simulink model "Virtual_Veh_Sim_EV3M_DLC"  (R2020a)
settings: configuration reference "Config_VarStep_Lat" (kept outside this file)
model workspace (MAT data in the model file):
  A = 159.22
  AccPwrbp = [0 0]
  AccSpdbp = [300 750]
  Aeff = 0.0314159265359
  Af = 2.46
  AfrStoich = 14.6
  AxlIxx = 62.3745166667
  AxlM = 160
  B = 1.01
  BattCapInit = 3.18
  BattCapInit_EV = 4.24
  BattChargeMax = 5.3
  BattChrgPwrMax = -60000
  BattChrgPwrMax_EV = -350000
  BattCurrMax = 300
  BattCurrMax_EV = 900
  BattDischrgPwrMax = 85000
  BattDischrgPwrMax_EV = 497000
  BattTempBp = [243.1 253.1 263.1 273.1 283.1 298.1 313.1]
  Battery.SOC_LUT = [0; 0.233616805137; 0.329414704495; 0.425212603853; 0.521010503211; 0.616808402569; 0.712606301927; 0.808404201284; 0.904202100642; 1]
  Battery.Temperature_LUT = [278.15 293.15 323.15]
  Battery.Capacity_LUT = [5.3 5.3 5.3]
  Battery.Em_LUT = [3.49587596064  3.51326111431  3.51592909009; 3.55858585798  3.5719535891  3.57237356974; 3.60724177033  3.62068327764  3.6276550187; 3.64771235788  3.65760001947  3.66611286097; 3.69314621195  3.69760962651  3.70681604299; 3.75549177279  3.75773263614  3.76696651763; 3.84165417727  3.85083489047  3.86645865382; 3.95105059257  3.95772489987  3.96617355496; 4.06366580695  4.067089232  4.07236317958; 4.1906518044  4.19061236732  4.19167206629]
  Battery.R0_LUT = [0.00999998116885  0.00969375106236  0.00708145896739; 0.00999856430024  0.00911239076326  0.00787358934878; 0.00998730272712  0.00894632530884  0.00837174615208; 0.00996262884044  0.00879430156772  0.00835611000801; 0.00987275439244  0.0083702809345  0.00820789809556; 0.00999543134051  0.00796657772792  0.0078372923375; 0.00990199705676  0.00829317762849  0.00843184907817; 0.00994753142013  0.00846223904615  0.00857747373973; 0.00988864262519  0.00860046339116  0.00783809261162; 0.00993546613466  0.00869430562795  0.00761030624168]
  Battery.R1_LUT = [0.00499947769959  0.00176414777168  0.00316403561543; 0.00499519961471  0.00182319958795  0.00222758288934; 0.00497942319098  0.00215602639557  0.00198515725158; 0.00498117211272  0.00190060293124  0.00183019810762; 0.00450940543796  0.0017898790503  0.00183803772559; 0.00398127966959  0.00191854781097  0.00207431379095; 0.00376691492773  0.00188008375757  0.00198672384849; 0.00419163622064  0.00214433717755  0.00161902199826; 0.00442604017912  0.00155246821646  0.0021103441137; 0.00431483823804  0.00154970784036  0.00218727749279]
  Battery.C1_LUT = [1983.38450838  78841.49366  1101.57625667; 4685.2948826  46429.6816213  4135.52830594; 9956.77541023  63356.4083796  12730.5976872; 11168.8695649  44437.7240428  12079.4670374; 4241.75396721  25121.8581323  9873.97196936; 4860.18499946  15430.1643159  2313.84302982; 8563.32887293  19567.7109152  8773.59604623; 11272.4596966  21732.1494006  11126.4679691; 3899.6527347  15798.9914071  2546.16773112; 2937.3854477  42171.3235856  1720.82916662]
  Battery.cell_mass = 0.066
  Battery.cell_rho_Cp = 2040000
  Battery.cell_Cp_heat = 964.92
  Battery.T_init = 288.15
  Battery.Qe_init = 1.06
  Battery.R_bleed = 20
  Battery.h_conv = 5
  Battery.cell_area = 0.1019
  Battery.TempInit = 298.15
  BrkPrsMax = 8273709
  Bx = 10
  C = 0.3618
  CapLUTBp = [0 0.01 0.02 0.03 0.04 0.05 0.06 0.07 0.08 0.09 0.1 0.11 0.12 0.13 0.14 0.15 0.16 0.17 0.18 0.19 0.2 0.21 0.22 0.23 0.24 0.25 0.26 0.27 0.28 0.29 0.3 0.31 0.32 0.33 0.34 0.35 0.36 0.37 0.38 0.39 0.4 0.41 0.42 0.43 0.44 0.45 0.46 0.47 0.48 0.49 0.5 0.51 0.52 0.53 0.54 0.55 0.56 0.57 0.58 0.59 0.6 0.61 0.62 0.63 0.64 0.65 0.66 0.67 0.68 0.69 0.7 0.71 0.72 0.73 0.74 0.75 0.76 0.77 0.78 0.79 0.8 0.81 0.82 0.83 0.84 0.85 0.86 0.87 0.88 0.89 0.9 0.91 0.92 0.93 0.94 0.95 0.96 0.97 0.98 0.99 1]
  CapSOCBp = [0 0.2 0.4 0.6 0.8 1]
  CatLightOffTime = 0
  Cd = 0.25
  ChrgLmt_bpt = [1 1 1 1 1 1 1 0.9 0.7 0.5 0]
  Cl = 0.1
  Cpm = 0.1
  Cps = 2
  CrankSpeed = 150
  Cx = 1.65
  Cz = 5565.2246438
  CzWhlAxl = 11490.971257
  DCT_Param.Transmission.Ratios = [3.78 2.18 1.43 1.03 0.935 0.84]
  DCT_Param.Transmission.Shaft_Inertia_Odd = 0.0023
  DCT_Param.Transmission.Shaft_Inertia_Even = 0.0009
  DCT_Param.Transmission.Shaft_Inertia_Output = 0.008
  DCT_Param.Transmission.Gear_Inertia = 0.001
  DCT_Param.Transmission.Gear_Efficiency = 0.94
  DCT_Param.Transmission.Gear_Ang_Vel_Thr = 0.01
  DCT_Param.Transmission.Shaft_Velocity_Odd = 0
  DCT_Param.Transmission.Shaft_Velocity_Even = 0
  DCT_Param.Transmission.Shaft_Velocity_Output = 0
  DCT_Param.Transmission.Gear_Initial_Velocity = 0
  DCT_Param.Transmission.Abstract.Compliance = 100000
  DCT_Param.Transmission.Abstract.Damping = 10000
  DCT_Param.Transmission.Abstract.Ratio_Time_Const = 0.05
  DCT_Param.Transmission.Abstract.Shift_Gear_Delay = 25
  DCT_Param.Clutch.Torque_Radius = 130
  DCT_Param.Clutch.Num_Friction_Surfaces = 4
  DCT_Param.Clutch.Engagement_Piston_Area = 0.001
  DCT_Param.Clutch.Kinetic_Friction_Coeff = 0.3
  DCT_Param.Clutch.Static_Friction_Coeff = 0.31
  DCT_Param.Clutch.Derating_Factor = 1
  DCT_Param.Clutch.Clutch_Velocity_Tolerance = 0.001
  DCT_Param.Clutch.Threshold_Pressure = 1
  DCT_Param.Clutch.Drag_Torque_Coeff = 0
  DCT_Param.Dog_Clutch.Max_Torque = 1000
  DCT_Param.Dog_Clutch.Teeth_Mean_Radius = 50
  DCT_Param.Dog_Clutch.Tooth_Height = 10
  DCT_Param.Dog_Clutch.Ring_Hub_Clearance = 3
  DCT_Param.Dog_Clutch.Ring_Stop_Stiffness = 1000000
  DCT_Param.Dog_Clutch.Ring_Stop_Damping = 1000
  DCT_Param.Dog_Clutch.Shift_Linkage_Damping = 100
  DCT_Param.Dog_Clutch.Max_Engage_Velocity = 1000000
  DCT_Param.Dog_Clutch.Tooth_Engage_Overlap = 3
  DCT_Param.Vehicle.Mass = 1600
  DCT_Param.Vehicle.Wheels_Per_Axle = 2
  DCT_Param.Vehicle.Distance_CG_FrontAxle = 1.7
  DCT_Param.Vehicle.Distance_CG_RearAxle = 2
  DCT_Param.Vehicle.Distance_CG_Ground = 0.5
  DCT_Param.Vehicle.Frontal_Area = 3
  DCT_Param.Vehicle.Aero_Drag_Coeff = 0.4
  DCT_Param.Vehicle.Initial_Velocity = 0
  DCT_Param.Vehicle.Final_Drive_Ratio = 3.7
  DCT_Param.Vehicle.Final_Drive_Efficiency = 0.86
  DCT_Param.Vehicle.Final_Drive_Vel_Thresh = 0.01
  DCT_Param.Vehicle.Side_Shaft_Inertia = 0.01
  DCT_Param.Vehicle.Side_Shaft_Initial_Velocity = 0
  DCT_Param.Vehicle.Tire.Radius = 0.312
  DCT_Param.Vehicle.Tire.Inertia = 0.5
  DCT_Param.Vehicle.Tire.Initial_Velocity = 0
  DCT_Param.Vehicle.Tire.Slip_Vel_Thresh = 0.1
  DCT_Param.Vehicle.Tire.Nominal_Vertical_Load = 4000
  DCT_Param.Vehicle.Tire.C_Coeff = 1.685
  DCT_Param.Vehicle.Tire.D_Coeff = [1.21 -0.037]
  DCT_Param.Vehicle.Tire.E_Coeff = [0.344 0.095 -0.02 0]
  DCT_Param.Vehicle.Tire.BCD_Coeff = [21.51 -0.163 0.245]
  DCT_Param.Vehicle.Tire.H_Coeff = [-0.002 0.002]
  DCT_Param.Vehicle.Tire.V_Coeff = [0 0]
  DCT_Param.ICE.Max_Power = 100000
  DCT_Param.ICE.Speed_At_Max_Power = 5500
  DCT_Param.ICE.Max_Speed = 7000
  DCT_Param.ICE.Stall_Speed = 200
  DCT_Param.ICE.Shaft_Inertia = 0.2
  DCT_Param.ICE.Initial_Velocity = 800
  DCT_Param.ICE.Idle_Ref_Spd = 800
  DCT_Param.ICE.Engine_Time_Constant = 0.2
  DCT_Param.ICE.Initial_Normalized_Throttle = 0
  DCT_Param.ICE.Speed_Threshold = 20
  DCT_Param.ICE.FC.Speed_Vector = [0 368.421052632 736.842105263 1105.26315789 1473.68421053 1842.10526316 2210.52631579 2578.94736842 2947.36842105 3315.78947368 3684.21052632 4052.63157895 4421.05263158 4789.47368421 5157.89473684 5526.31578947 5894.73684211 6263.15789474 6631.57894737 7000]
  DCT_Param.ICE.FC.Torque_Vector = [0 10.5263157895 21.0526315789 31.5789473684 42.1052631579 52.6315789474 63.1578947368 73.6842105263 84.2105263158 94.7368421053 105.263157895 115.789473684 126.315789474 136.842105263 147.368421053 157.894736842 168.421052632 178.947368421 189.473684211 200]
  DCT_Param.ICE.FC.Consumption_Table = [0.262945178015 0.225304787522 0.201465019624 0.191425874321 0.195187351614 0.212749451502 0.244112173984 0.289275519063 0.348239486736 0.421004077004 0.507569289868 0.607935125326 ... (400 elements, 20x20)]
  DCT_Param.Shift_Map_Example.Pedal_Positions = [0.1 0.4 0.5 0.9]
  DCT_Param.Shift_Map_Example.Upshift_Speeds = [11  20  26  34.5  43; 14  26  35  44.5  55; 17  31  42  52.5  65; 21  39  52  66.5  80]
  DCT_Param.Shift_Map_Example.Downshift_Speeds = [8.9  17  23.6  32.4  40.8; 11.5  22.7  32  41.6  52.2; 14  27  38.1  50  62; 18  33  48  62.6  76.2]
  DCT_Param.Shift_Map_ORIG.Pedal_Positions = [0.1 0.4 0.5 0.9]
  DCT_Param.Shift_Map_ORIG.Upshift_Speeds = [11.5  23.5  35.5  45.5  55.5; 14.5  26.5  38.5  48.5  58.5; 17.5  29.5  41.5  51.5  61.5; 20.5  32.5  44.5  54.5  64.5]
  DCT_Param.Shift_Map_ORIG.Downshift_Speeds = [8.5  20.5  32.5  42.5  52.5; 11.5  23.5  35.5  45.5  55.5; 14.5  26.5  38.5  48.5  58.5; 17.5  29.5  41.5  51.5  61.5]
  DCT_Param.Shift_Map_OPT.Pedal_Positions = [0.1 0.4 0.5 0.9]
  DCT_Param.Shift_Map_OPT.Upshift_Speeds = [17.8469  29.8469  35.8159  41.2981  46.3004; 19.2469  33.9778  43.9778  53.9778  63.9778; 24.5469  41.9778  62.1778  78.5778  106.9778; 27.5469  59.3778  99.0445  109.0445  119.0445]
  DCT_Param.Shift_Map_OPT.Downshift_Speeds = [14.8469  26.8469  32.8159  38.2981  43.3004; 16.2469  30.9778  40.9778  50.9778  60.9778; 21.5469  38.9778  59.1778  75.5778  103.9778; 24.5469  56.3778  96.0445  106.0445  116.0445]
  DCT_Param.Shift_Map.Pedal_Positions = [0.1 0.4 0.5 0.9]
  DCT_Param.Shift_Map.Upshift_Speeds = [11.5  23.5  35.5  45.5  55.5; 14.5  26.5  38.5  48.5  58.5; 17.5  29.5  41.5  51.5  61.5; 20.5  32.5  44.5  54.5  64.5]
  DCT_Param.Shift_Map.Downshift_Speeds = [8.5  20.5  32.5  42.5  52.5; 11.5  23.5  35.5  45.5  55.5; 14.5  26.5  38.5  48.5  58.5; 17.5  29.5  41.5  51.5  61.5]
  DCT_Param.Control.Clutch.Min_Lock_Pressure = 2000000
  DCT_Param.Control.Clutch.Max_Lock_Pressure = 5000000
  DCT_Param.Control.Clutch.Max_Unlock_Pressure = 500000
  DCT_Param.Control.Engine_Start_RPM = 800
  DCT_Param.Control.Engine_Stop_RPM = 790
  DCT_Param.Control.Mode_Logic_TS = 0.1
  DCT_Param.Control.ICE.Kp = 0.02
  DCT_Param.Control.ICE.Ki = 0.01
  DCT_Param.Control.Gen.Kp = 10
  DCT_Param.Control.Gen.Ki = 3
  DCT_Param.Control.Mot.Kp = 500
  DCT_Param.Control.Mot.Ki = 300
  DCT_Param.Control.Veh_Spd.Kp = 0.02
  DCT_Param.Control.Veh_Spd.Ki = 0.04
  DCT_Param.Driver.Kp = 400
  DCT_Param.Driver.Ki = 0.001
  DCT_Param.Driver.Pedal_Filter_Const = 0.01
  DCT_Param.Dog_Clutches.Pulse_Delay = 50
  DCT_Param.Dog_Clutches.Pulse_Length = 20
  DCT_Param.Animation.Teeth_Ratios = [0.338461538462 0.555555555556 0.916666666667 0.96 1.17948717949 1.92307692308]
  DCT_Param.Animation.Teeth_Ratios_Reverse = [0.458333333333 0.75]
  DCT_Param.Shift_Map_OPT506.Pedal_Positions = [0.1 0.4 0.5 0.9]
  DCT_Param.Shift_Map_OPT506.Upshift_Speeds = [18  30.2  48.3  67.3322  77.3429; 20.1  36.85  66.6178  76.7537  86.7537; 21.1  40.25  71.0189  81.0189  91.7873; 24.1  63.75  80.7523  105.9489  115.9489]
  DCT_Param.Shift_Map_OPT506.Downshift_Speeds = [15  27.2  45.3  64.3322  74.3429; 17.1  33.85  63.6178  73.7537  83.7537; 18.1  37.25  68.0189  78.0189  88.7873; 21.1  60.75  77.7523  102.9489  112.9489]
  DCT_Param.Shift_Map_OPTAbsRea176.Pedal_Positions = [0.1 0.4 0.5 0.9]
  DCT_Param.Shift_Map_OPTAbsRea176.Upshift_Speeds = [17.8469  29.8469  35.7875  44.0901  49.4243; 18.9219  34.1312  45.8256  59.7585  69.7585; 32.1719  43.4585  53.51  103.2151  114.6401; 35.1719  59.2585  99.5217  109.5217  119.5217]
  DCT_Param.Shift_Map_OPTAbsRea176.Downshift_Speeds = [14.8469  26.8469  32.7875  41.0901  46.4243; 15.9219  31.1312  42.8256  56.7585  66.7585; 29.1719  40.4585  50.51  100.2151  111.6401; 32.1719  56.2585  96.5217  106.5217  116.5217]
  DischrgLmt_bpt = [0 0.5 0.7 0.9 1 1 1 1 1 1 1]
  Dn_Shft_Spd = [3  7  11  15  19; 3  7  11  15  19; 10  17  26  35  49; 10  17  26  35  49]
  Downshift_Speeds = [9.5625  23.0625  36.5625  47.8125  59.0625  68.90625  78.75; 12.9375  26.4375  39.9375  51.1875  62.4375  72.84375  83.25; 16.3125  29.8125  43.3125  54.5625  65.8125  76.78125  87.75; 19.6875  33.1875  46.6875  57.9375  69.1875  80.71875  92.25]
  Dx = 1
  ECMS_Ki = 0.1
  ECMS_Kp = 3
  ECMS_method = 1
  ECMS_s = 3.4
  Em = [2.8 3.228 3.284 3.361 3.408 3.427 3.472 3.477 3.493 3.504 3.516 3.528 3.537 3.545 3.555 3.561 3.566 3.576 3.587 3.589 3.594 3.6 3.608 3.61 3.616 3.619 3.626 3.632 3.637 3.64 3.645 3.646 3.652 3.655 3.658 3.661 3.664 3.668 3.673 3.678 3.68 3.681 3.686 3.692 3.699 3.702 3.705 3.71 3.717 3.723 3.728 3.733 3.735 3.742 3.749 3.755 3.761 3.768 3.773 3.78 3.791 3.798 3.798 3.814 3.818 3.825 3.841 3.846 3.855 3.863 3.877 3.885 3.894 3.907 3.919 3.926 3.935 3.944 3.954 3.964 3.974 3.988 3.998 4.014 4.029 4.034 4.047 4.065 4.074 4.086 4.097 4.131 4.126 4.138 4.15 4.18 4.174 4.187 4.207 4.231 4.221]
  EngStopStartEnable = 1
  EngStopTime = Simulink.Parameter
  EngStopTime.Value = 0
  EngStopTime.DataType = 'auto'
  EngStopTime.Dimensions = [1 1]
  EngTrqCmd_0 = [0 5.91462851599 6.30130128159 6.63745773103 6.93103920513 7.1887141028 7.41614736865 7.6182009157 7.79908238179 7.96245469721 8.11151569725 8.24905488129 8.37749301819 8.49890935932 8.61506054978 8.72739478049 8.8370641951 8.94493799505 9.05161804887 9.15745812086 9.26258713198]
  Ex = 0.01
  F0z = [2886 2907]
  F0zWhlAxl = 2907
  FZMAX = 6570
  FZMIN = 0
  Fc = 500
  FsbF = [-700000 -7000 -700 0 700 7000 700000]
  FsbR = [-700000 -7000 -700 0 700 7000 700000]
  FskF = [-8928.57142857 -178.571428571 0 357.142857143 535.714285714 9285.71428571]
  FskR = [-5357.14285714 -107.142857143 0 214.285714286 321.428571429 5571.42857143]
  G = [-1 0 1 2 3 4 5 6]
  G_o = 1
  Gear_Dn_bpt = [2 3 4 5 6]
  Gear_Up_bpt = [1 2 3 4 5]
  HEVEngTrq_min = 16.186104388
  Hmax = 0.25
  Iyy = 3000
  Iyy_Whl = 0.8
  J = 0.01
  J1 = 0.01
  J2 = 0.01
  Jd = 0.025
  Ji = 0.1
  Jin = 0.05
  Jin_Cltch = 0.2
  Jin_Cltch2 = 0.01
  Jout = [0.01 0.009 0.01 0.01 0.01 0.01 0.01 0.01]
  Jout_Cltch = 0.01
  Jout_Cltch2 = 0.05
  Jt = 0.1
  Jw1 = 0.01
  Jw2 = 0.01
  K_c = 10000
  Kpt = 12798
  Kz = 52451.0065793
  KzWhlAxl = 138031.612078
  LHV = 43000000
  Lhv = 42940000
  Lrel = 0.15
  Mass = 1623
  MaxTorque = [10.8721902117; 76.2227873944; 95.7133163788; 115.203846226; 134.694376076; 154.184905918; 173.675435766; 181.839920951; 181.509869828; 181.17981871; 180.849767971; 180.519716854; 180.189665737; 179.859612653; 179.529561534; 179.199510415; 178.869460888; 178.539409771; 178.209357061; 177.879307536; 177.549246888]
  N = [3.39 1 4.212 2.637 1.8 1.386 1 0.772]
  NCyl = 4
  NF = 2
  NR = 2
  N_P0 = 3
  N_P4 = 4.1
  N_idle = 750
  Ndiff = 3.32
  Ndiff_P4 = 4.1
  Ndiff_front = 5
  Ndiff_rear = 3.5
  Ndisk = 1
  Ndisks = 4
  Ngrid = 200
  Np = 2
  Np_EV = 35
  Np_FC = 1
  Ns = 72
  Ns_EV = 96
  Pabs = 101325
  Pdl_Pos_Dn_bpt = [0 0.6 0.9 1]
  Pdl_Pos_Up_bpt = [0 0.25 0.9 1]
  Pedal_Positions = [0.1 0.4 0.5 0.9]
  PenaltyFctr = 10000000
  Plimit = 60000
  Plimit_EV = 350000
  Press = 7000000
  Pstd = 101325
  RInt = [0.008846  0.009319  0.009027  0.00847  0.01032  0.01314; 0.006389  0.006554  0.005553  0.005525  0.006043  0.007805; 0.004364  0.004101  0.00406  0.003452  0.003846  0.004517; 0.002031  0.002563  0.002532  0.00246  0.002716  0.003047; 0.001443  0.001825  0.001795  0.001778  0.001924  0.002234; 0.0005603  0.0007192  0.0006887  0.0007557  0.0007355  0.001014; 0.001028  0.001338  0.001  0.001536  0.001546  0.002789]
  Rair = 287
  Re = 0.327
  Reff = 0.11
  Reff_LSD = 0.2
  RegenBrkCutOff = [0 1]
  RegenBrkSpd_bpt = [2.2352 4.4704]
  Rm = 0.15
  SOCInit = 0.5
  SOCTrgt = 60
  SOC_bpt = [0 0.1 0.2 0.3 0.4 0.5 0.6 0.7 0.8 0.9 1]
  SOCmax = 80
  SOCmin = 40
  SUS.Zeta = 0.7071
  SUS.Wd = 9.42477796077
  SUS.Stiffness = 52451.0065793
  SUS.Damping.Constant = 5565.2246438
  SUS.UnsprungMass.Fr = 21.0693333333
  SUS.UnsprungMass.Rr = 21.0693333333
  Sg = 0.743
  Sinj = 6.45161290323
  T = 273
  TCopy = 300
  T_eff_bp = [0 20 40 60 80 100 120 140 160 180 200]
  T_eff_bp_EV_front = [0 30 60 90 120 150 180 210 240 270 300]
  T_eff_bp_EV_rear = [0 20 40 60 80 100 120 140 160 180 200]
  T_eff_bp_P0 = [0 5.78745247607 6.36619772368 7.07355302631 7.95774715459 9.09456817668 10.6103295395 12.7323954474 15.9154943092 21.2206590789 66.6666666667]
  T_init = 298.15
  T_t = [200 200 200 200 190.9859317 143.2394488 114.591559 95.49296586 81.85111359 71.61972439 63.66197724 57.29577951 52.08707228 47.74648293]
  T_t_EV_front = [300 300 300 300 286.47889755 214.8591732 171.8873385 143.23944879 122.776670385 107.429586585 95.49296586 85.943669265 78.13060842 71.619724395]
  T_t_EV_rear = [200 200 200 200 190.9859317 143.2394488 114.591559 95.49296586 81.85111359 71.61972439 63.66197724 57.29577951 52.08707228 47.74648293]
  T_t_P0 = [66.6666666667 66.6666666667 66.6666666667 66.6666666667 21.2206590789 15.9154943092 12.7323954474 10.6103295395 9.09456817668 7.95774715459 7.07355302631 6.36619772368 5.78745247607 5.30516476973]
  Tc_Batt = 0.001
  Tc_DC = 0.001
  Tc_Mot = 0.02
  Temp_bpts = [313 358]
  TimeCnstECP = 0.125
  TimeCnstEGR = 0.125
  TimeCnstETC = 0.085
  TimeCnstICP = 0.125
  TimeCnstIVL = 0.125
  TimeCnstMFA = 0.125
  TimeCnstSWVA = 0.125
  TimeCnstVCR = 0.125
  TimeCnstVGT = 0.15
  TimeCnstVIRL = 0.125
  TimeCnstWGA = 0.15
  TimeStep = 0.0001
  TracPenaltyFctr = 50
  Trans.InputShaftInertia = 0.01
  Trans.InputShaftDamping = 0.001
  Trans.FinalDrive = 2.77
  Trans.GearRatios = [-3.82 4.56 4.56 2.97 2.08 1.69 1.27 1 0.85 0.65]
  Trans.GearNums = [-1 0 1 2 3 4 5 6 7 8]
  Trans.Inertias = [0.128 0.01 0.128 0.1 0.062 0.028 0.01 0.01 0.01 0.01]
  Trans.DampingCoeffs = [0.003 0.001 0.003 0.0025 0.002 0.001 0.001 0.001 0.001 0.001]
  Trans.Efficiencies = [0.9 0.9 0.9 0.9 0.9 0.95 0.95 0.95 0.95 0.95]
  Trans.ShiftTau = 0.01
  Trq_bpts = [25 50 75 100 150 200 250]
  Ts = Simulink.Parameter
  Ts.Value = 0.01
  Ts.DataType = 'auto'
  Ts.Dimensions = [1 1]
  Tstd = 293.15
  UNLOADED_RADIUS = 0.336
  Up_Shft_Spd = [5  9  13  17  21; 5  9  13  17  21; 12  19  28  37  51; 12  19  28  37  51]
  Upshift_Speeds = [12.9375  26.4375  39.9375  51.1875  62.4375  72.84375  83.25; 16.3125  29.8125  43.3125  54.5625  65.8125  76.78125  87.75; 19.6875  33.1875  46.6875  57.9375  69.1875  80.71875  92.25; 33  52.5  77.25  100.5  138.75  161.875  185]
  VEH.Mass = 1181
  VEH.StaticNormalFrontLoad.FR = 264.666666667
  VEH.StaticNormalFrontLoad.FL = 264.666666667
  VEH.StaticNormalRearLoad.RR = 322
  VEH.StaticNormalRearLoad.RL = 322
  VEH.WheelBase = 3.075
  VEH.FrontAxlePositionfromCG = 1.515
  VEH.RearAxlePositionfromCG = 1.504
  VEH.HeightCG = 0.134
  VEH.FrontalArea = 2.11
  VEH.DragCoefficient = 0.33
  VEH.NumberOfWheelsPerAxle = 2
  VEH.Thread.FR = 1.705
  VEH.Thread.RR = 1.705
  VEH.PitchMomentInertia = 1922.66666667
  VEH.RollMomentInertia = 432.333333333
  VEH.YawMomentInertia = 2066
  VEH.SteeringRatio = 18
  VEH.TrackWidth = 1.922
  VEH.SprungMass = 1096.72266667
  VEH.InitialLongPosition = 0
  VEH.InitialLatPosition = 3.125
  VEH.InitialVertPosition = 0
  VEH.InitialRollAngle = 0
  VEH.InitialPitchAngle = 0
  VEH.InitialYawAngle = 0
  VEH.InitialLongVel = 0
  VEH.InitialLatVel = 0
  VEH.InitialVertVel = 0
  VEH.InitialRollRate = 0
  VEH.InitialPitchRate = 0
  VEH.InitialYawRate = 0
  VXLOW = 2
  Vd = 0.0015
  Vinit = 650
  WH.Mass = 11.4333333333
  a = 3
  aMy = 0.01
  a_CG = 1.09
  afr_stoich = 14.6
  alphaMy = 0
  b = Simulink.Parameter
  b.Value = 1000
  b.DataType = 'auto'
  b.Dimensions = [1 1]
  b1 = 100
  b1_g = 0.001
  b2 = 100
  b2_g = 0.001
  bMy = 0
  b_CG = 1.7
  b_J = 0.001
  bd = 0.001
  behavior = 0.2
  betaMy = 1
  bi = 0.001
  bin = 0.003
  bin_Cltch = 0.003
  bout = [0.003 0.003 0.003 0.003 0.003 0.003 0.003 0.003]
  bout_Cltch = 0.003
  br = 0.001
  bt = 0.001
  bw1 = 0.001
  bw2 = 0.001
  cMy = 0
  controller_type = 2
  defaultSpacing = 15
  disk_abore = 0.05
  domega_o = 0
  dt3D = 0.05
  dw = [0 10 20 40 60 80 100]
  dzdotsF = [-10 -1 -0.1 0 0.1 1 10]
  dzdotsR = [-10 -1 -0.1 0 0.1 1 10]
  dzsF = [-0.005 -0.0001 0 0.2 0.2001 0.2051]
  dzsR = [-0.005 -0.0001 0 0.2 0.2001 0.2051]
  eff = 98
  efficiency_table = [52  78  80  82  82  80  78  78  76  74  70; 52  78  80  82  82  80  78  78  76  74  70; 52  78  84  86  86  86  86  84  84  82  82; 52  80  86  86  88  88  88  86  86  84  84; 52  80  86  88  88  88  88  88  86  86  86; 52  80  86  88  90  90  90  90  88  88  88; 52  82  88  90  91  91  92  92  92  91  91; 52  82  88  91  91  92  93  93  93  93  93; 52  84  90  92  92  93  93  93  93  93  93; 62  86  91  93  93  93  93  93  93  93  93; 66  86  91  93  93  93  93  93  93  93  93; 70  86  92  93  93  93  93  93  93  93  93; 70  86  92  93  93  93  93  93  93  93  93; 72  86  91  93  93  93  93  93  93  93  93]
  efficiency_table_EV = [85  85  85  85  85  85  85  85  85  85  85; 85  85  90  90  90  90  90  90  90  90  88; 85  85  92  92  92  92  92  92  92  92  92; 85  85  92  92  93  93  93  93  92  92  92; 85  85  93  94  94  94  94  94  94  94  94; 85  85  93  94  94  95  95  95  95  95  95; 85  85  93  94  94  95  95  95  95  95  95; 85  85  93  94  95  95  95  95  95  95  95; 85  85  93  94  95  95  95  95  95  95  95; 85  85  93  94  94  94  94  94  94  94  94; 85  85  90  92  93  93  93  93  93  93  93; 85  85  90  92  93  93  93  93  93  93  93; 85  85  90  92  93  93  93  93  93  93  93; 85  85  90  92  93  93  93  93  93  93  93]
  efficiency_table_P0 = [52  78  80  82  82  80  78  78  76  74  70; 52  78  80  82  82  80  78  78  76  74  70; 52  78  84  86  86  86  86  84  84  82  82; 52  80  86  86  88  88  88  86  86  84  84; 52  80  86  88  88  88  88  88  86  86  86; 52  80  86  88  90  90  90  90  88  88  88; 52  82  88  90  91  91  92  92  92  91  91; 52  82  88  91  91  92  93  93  93  93  93; 52  84  90  92  92  93  93  93  93  93  93; 62  86  91  93  93  93  93  93  93  93  93; 66  86  91  93  93  93  93  93  93  93  93; 70  86  92  93  93  93  93  93  93  93  93; 70  86  92  93  93  93  93  93  93  93  93; 72  86  91  93  93  93  93  93  93  93  93]
  egotf = tf
  egotf.IOSize_ = [1 1]
  egotf.Data_ = ltipack.tfdata
  egotf.Data_.num = {[0 0 1]}
  egotf.Data_.den = {[0.5 1 0]}
  egotf.Data_.Delay.Input = 0
  egotf.Data_.Delay.Output = 0
  egotf.Data_.Delay.IO = 0
  egotf.Data_.Ts = 0
  elec_Pipe.Length = 75
  elec_Pipe.Dh = 2.5
  elec_Pipe.Area = 4.90873852123
  elec_Radiator.AreaG = 0.15
  elec_Radiator.VolumeG = 0.01
  elec_Radiator.AreaL = 0.000314159265359
  elec_Radiator.VolumeL = 0.000157079632679
  elec_Radiator.mdotG = [0.1 8]
  elec_Radiator.mdotL = [0.1 5]
  elec_Radiator.SD = [1  9; 2  10]
  elec_Radiator.dPG = [0.003 0.01]
  elec_Radiator.dPL = [0.005 0.02]
  eta = [0.95 0.95 0.95 0.95 0.95 0.95 0.95 0.95]
  eta_tbl = [0.7 0.8 0.9 0.9 0.9 0.9 0.9 0.7 0.8 0.9 0.9 0.9 ... (1232 elements, 7x11x8x2)]
  f_air = [0 0 0 0 0 0 0 0 0 0 0 0 ... (441 elements, 21x21)]
  f_co = [0 0 0 0 0 0 0 0 0 0 0 0 ... (441 elements, 21x21)]
  f_co2 = [0 0 0 0 0 0 0 0 0 0 0 0 ... (441 elements, 21x21)]
  f_cp_ld_bpt = [0 0.2 0.275 0.35 0.425 0.5 0.575 0.65 0.725 0.8 0.875 0.95 1.025 1.1 1.175 1.25]
  f_cp_n_bpt = [750 1053.57142857 1357.14285714 1660.71428571 1964.28571429 2267.85714286 2571.42857143 2875 3178.57142857 3482.14285714 3785.71428571 4089.28571429 4392.85714286 4696.42857143 5000]
  f_del_sa_bpt = [0 0.75 1.5 2.25 3 3.75 4.5 5.25 6 6.75 7.5 8.25 9 9.75 10.5 11.25 12 12.75 13.5 14.25 15 15.75 16.5 17.25 18 18.75 19.5 20.25 21 21.75 22.5 23.25 24 24.75 25.5 26.25 27 27.75 28.5 29.25 30 30.75 31.5 32.25 33 33.75 34.5 35.25 36 36.75 37.5 38.25 39 39.75 40.5 41.25 42 42.75 43.5 44.25 45 45.75 46.5 47.25 48]
  f_ecp = [0 0 7.19012817097 15.3709456879 19.1470470057 19.0854874367 13.5819971805 0 0 0 0 0 ... (240 elements, 16x15)]
  f_eff = [499.877436556 432.508206156 399.540781628 370.894662993 347.954880181 331.11554878 319.468905906 311.408898718 305.523567029 300.961538912 297.204959405 293.79866205 ... (441 elements, 21x21)]
  f_egr_areapct_cmd = [0 3.448 6.897 10.34 13.79 17.24 20.69 24.14 27.59 31.03 34.48 37.93 ... (600 elements, 30x20)]
  f_egr_areapct_nrmlzdflow_bpt = [0 0.03448 0.06897 0.1034 0.1379 0.1724 0.2069 0.2414 0.2759 0.3103 0.3448 0.3793 0.4138 0.4483 0.4828 0.5172 0.5517 0.5862 0.6207 0.6552 0.6897 0.7241 0.7586 0.7931 0.8276 0.8621 0.8966 0.931 0.9655 1]
  f_egr_areapct_pr_bpt = [0.5; 0.5263; 0.5526; 0.5789; 0.6053; 0.6316; 0.6579; 0.6842; 0.7105; 0.7368; 0.7632; 0.7895; 0.8158; 0.8421; 0.8684; 0.8947; 0.9211; 0.9474; 0.9737; 1]
  f_egr_max_stdflow = [74.87 74.87 74.74 74.39 73.81 72.98 71.91 70.58 68.97 67.06 64.84 62.25 59.27 55.81 51.79 47.07 36.33 24.22 12.11 0]
  f_egr_stdflow = [0 3.743 7.487 11.23 14.97 18.72 22.46 26.2 29.95 33.69 37.43 41.18 ... (420 elements, 21x20)]
  f_egr_stdflow_egrap_bpt = [0; 5; 10; 15; 20; 25; 30; 35; 40; 45; 50; 55; 60; 65; 70; 75; 80; 85; 90; 95; 100]
  f_egr_stdflow_pr_bpt = [0.5; 0.5263; 0.5526; 0.5789; 0.6053; 0.6316; 0.6579; 0.6842; 0.7105; 0.7368; 0.7632; 0.7895; 0.8158; 0.8421; 0.8684; 0.8947; 0.9211; 0.9474; 0.9737; 1]
  f_egrpct_cmd = [0  0  0  0  0  0  0  0  0  0  0  0  0  0  0; 0  0  0  0  0  0  0  0  0  0  0  0  0  0  0; 0  0  0  0  0  0  0  0  0  0  0  0  0  0  0; 0  0  0  0  0  0  0  0  0  0  0  0  0  0  0; 0  0  0  0  0  0  0  0  0  0  0  0  0  0  0; 0  0  0  0  0  0  0  0  0  0  0  0  0  0  0; 0  0  0  0  0  0  0  0  0  0  0  0  0  0  0; 0  0  0  0  0  0  0  0  0  0  0  0  0  0  0; 0  0  0  0  0  0  0  0  0  0  0  0  0  0  0; 0  0  0  0  0  0  0  0  0  0  0  0  0  0  0; 0  0  0  0  0  0  0  0  0  0  0  0  0  0  0; 0  0  0  0  0  0  0  0  0  0  0  0  0  0  0; 0  0  0  0  0  0  0  0  0  0  0  0  0  0  0; 0  0  0  0  0  0  0  0  0  0  0  0  0  0  0; 0  0  0  0  0  0  0  0  0  0  0  0  0  0  0; 0  0  0  0  0  0  0  0  0  0  0  0  0  0  0]
  f_egrpct_ld_bpt = [0 0.2 0.275 0.35 0.425 0.5 0.575 0.65 0.725 0.8 0.875 0.95 1.025 1.1 1.175 1.25]
  f_egrpct_n_bpt = [750 1054 1357 1661 1964 2268 2571 2875 3179 3482 3786 4089 4393 4696 5000]
  f_fric_temp_bpt = [275 277 279 281 283 285 287 289 291 293 295 297 299 301 303 305 307 309 311 313 315 317 319 321 323 325 327 329 331 333 335 337 339 341 343 345 347 349 351 353 355 357 359 361 363 365]
  f_fric_temp_mod = [3.986 2.616 2.132 1.946 1.839 1.747 1.672 1.608 1.551 1.499 1.462 1.415 1.363 1.314 1.275 1.248 1.223 1.195 1.173 1.15 1.134 1.113 1.097 1.082 1.065 1.051 1.039 1.025 1.01 1.001 0.9907 0.9802 0.9699 0.9595 0.9593 0.954 0.9415 0.9368 0.9285 0.923 0.9185 0.9093 0.9018 0.8989 0.8965 0.887]
  f_fuel = [0 0 0 0 0 0 0 0 0 0 0 0 ... (441 elements, 21x21)]
  f_hc = [0 0 0 0 0 0 0 0 0 0 0 0 ... (441 elements, 21x21)]
  f_icp = [0 0 1 1.09273642197 2.29409401139 3.54274371837 0.947749647567 0 0 0 0 0 ... (240 elements, 16x15)]
  f_intksys_stdflow_bpt = [0 29.67 59.34 89.01 117.8 144.1 155.7 166 175.2 183.3 190.7 197 202.7 207.7 212.2 216.1 219.4 222.2 224.5 226.4]
  f_intksys_stdflow_pr = [1 0.9789 0.9579 0.9368 0.9158 0.8947 0.8737 0.8526 0.8316 0.8105 0.7895 0.7684 0.7474 0.7263 0.7053 0.6842 0.6632 0.6421 0.6211 0.6]
  f_lamcmd = [1  1  1  1  1  1  1  1  1  1  1  1  1  1  1; 1  1  1  1  1  1  1  1  1  1  1  1  1  1  1; 1  1  1  1  1  1  1  1  1  1  1  1  1  1  1; 1  1  1  1  1  1  1  1  1  1  1  1  1  1  1; 1  1  1  1  1  1  1  1  1  1  1  1  1  1  1; 1  1  1  1  1  1  1  1  1  1  1  1  1  1  1; 1  1  1  1  1  1  1  1  1  1  1  1  1  1  1; 1  1  1  1  1  1  1  1  1  1  1  1  1  1  1; 1  1  1  1  1  1  1  1  1  1  1  1  1  1  1; 1  1  1  1  1  1  1  1  1  1  1  1  1  1  1; 1  1  1  1  1  1  1  1  1  1  1  1  1  1  0.978833376279; 1  1  1  1  1  0.994115442909  1  0.972947102204  0.980523305065  0.999379925377  1  0.999606769395  0.999730304812  0.995941175028  0.966904774685; 1  1  1  0.94651624294  1  0.952506105741  0.994491417815  0.906466250495  0.924122061249  0.974767007025  0.985748891861  0.982416523617  0.992900047913  0.942109771144  0.941787575943; 1  1  1  0.942  0.937279637266  0.910896768573  0.929830385386  0.839985398785  0.854904769548  0.889462296842  0.92380217143  0.919912974116  0.958707785886  0.945711085936  0.914402970615; 1  1  1  0.942  0.902  0.869287431405  0.865169352957  0.81  0.824  0.812  0.837314196571  0.85940898562  0.888506841156  0.882667105929  0.87548189152; 1  1  1  0.942  0.902  0.846  0.824  0.81  0.824  0.812  0.826  0.818  0.815209011399  0.813810193086  0.836]
  f_lamcmd_ld_bpt = [0 0.2 0.275 0.35 0.425 0.5 0.575 0.65 0.725 0.8 0.875 0.95 1.025 1.1 1.175 1.25]
  f_lamcmd_n_bpt = [750 1053.57142857 1357.14285714 1660.71428571 1964.28571429 2267.85714286 2571.42857143 2875 3178.57142857 3482.14285714 3785.71428571 4089.28571429 4392.85714286 4696.42857143 5000]
  f_lcmd = [0 0.323404450126 0.402272754123 0.472190900601 0.545782048677 0.619112163094 0.619299299836 0.619299299836 0.619299299836 0.619299299836 0.619299299836 0.619299299836 ... (315 elements, 21x15)]
  f_lcmd_n_bpt = [750 1053.57142857 1357.14285714 1660.71428571 1964.28571429 2267.85714286 2571.42857143 2875 3178.57142857 3482.14285714 3785.71428571 4089.28571429 4392.85714286 4696.42857143 5000]
  f_lcmd_tq_bpt = [0 15 25.2631578947 35.5263157895 45.7894736842 56.0526315789 66.3157894737 76.5789473684 86.8421052632 97.1052631579 107.368421053 117.631578947 127.894736842 138.157894737 148.421052632 158.684210526 168.947368421 179.210526316 189.473684211 199.736842105 210]
  f_m_lam = [0.94128 0.95565 0.97001 0.98437 0.99008 1.0004 0.97527 0.9549 0.92612 0.89735]
  f_m_lam_bpt = [0.65 0.7 0.75 0.8 0.85 0.9 0.95 1 1.05 1.1]
  f_m_sa = [1.0019 0.9988 0.9953 0.99173 0.98811 0.98441 0.98065 0.97682 0.97293 0.96897 0.96493 0.96083 0.95666 0.95242 0.94811 0.94373 0.93927 0.93475 0.93015 0.92548 0.92074 0.91592 0.91104 0.90608 0.90105 0.89594 0.89076 0.88551 0.88019 0.8748 0.86933 0.86379 0.85818 0.8525 0.84675 0.84093 0.83503 0.82907 0.82303 0.81693 0.81075 0.80451 0.79819 0.79181 0.78536 0.77884 0.77226 0.7656 0.75888 0.75209 0.74524 0.73832 0.73134 0.72429 0.71717 0.70999 0.70275 0.69682 0.68949 0.68303 0.67548 0.67037 0.66525 0.66014 0.65503]
  f_mdot_air_corr = [1.02156051768 1.00597426471 0.989411677851 1.0033499089 0.984591437857 0.988509040623 1.0326198627 1.02765527362 1.0134784519 0.998280021213 0.981755128787 0.967218261288 ... (400 elements, 20x20)]
  f_mdot_air_corr_ld_bpt = [0.223381333333 0.285105122807 0.346828912281 0.408552701754 0.470276491228 0.532000280702 0.593724070175 0.655447859649 0.717171649123 0.778895438596 0.84061922807 0.902343017544 0.964066807018 1.02579059649 1.08751438596 1.14923817544 1.21096196491 1.27268575439 1.33440954386 1.39613333333]
  f_mdot_air_n_bpt = [750 973.6842 1197.3684 1421.0526 1644.7368 1868.4211 2092.1053 2315.7895 2539.4737 2763.1579 2986.8421 3210.5263 3434.2105 3657.8947 3881.5789 4105.2632 4328.9474 4552.6316 4776.3158 5000]
  f_mdot_intk = [0 0 0 0 0 0 0 0 0 0 0 0 ... (400 elements, 20x20)]
  f_mdot_intk_ecp_bpt = [0 2.6316 5.2632 7.8947 10.5263 13.1579 15.7895 18.4211 21.0526 23.6842 26.3158 28.9474 31.5789 34.2105 36.8421 39.4737 42.1053 44.7368 47.3684 50]
  f_mdot_trpd_bpt = [0 5.7895 11.5789 17.3684 23.1579 28.9474 34.7368 40.5263 46.3158 52.1053 57.8947 63.6842 69.4737 75.2632 81.0526 86.8421 92.6316 98.4211 104.2105 110]
  f_nox = [0 0 0 0 0 0 0 0 0 0 0 0 ... (441 elements, 21x21)]
  f_nv = [0.64175366561 0.641419295169 0.640125365558 0.638690556197 0.644169906538 0.669178791311 0.731659452876 0.750078238889 0.750078238889 0.750078238889 0.750078238889 0.750078238889 ... (225 elements, 15x15)]
  f_nv_n_bpt = [750 1053.57142857 1357.14285714 1660.71428571 1964.28571429 2267.85714286 2571.42857143 2875 3178.57142857 3482.14285714 3785.71428571 4089.28571429 4392.85714286 4696.42857143 5000]
  f_nv_prs_bpt = [31 40.6428571429 50.2857142857 59.9285714286 69.5714285714 79.2142857143 88.8571428571 98.5 108.142857143 117.785714286 127.428571429 137.071428571 146.714285714 156.357142857 166]
  f_pm = [0  0  0  0  0  0  0  0  0  0  0  0  0  0  0  0  0  0  0  0  0; 0  0  0  0  0  0  0  0  0  0  0  0  0  0  0  0  0  0  0  0  0; 0  0  0  0  0  0  0  0  0  0  0  0  0  0  0  0  0  0  0  0  0; 0  0  0  0  0  0  0  0  0  0  0  0  0  0  0  0  0  0  0  0  0; 0  0  0  0  0  0  0  0  0  0  0  0  0  0  0  0  0  0  0  0  0; 0  0  0  0  0  0  0  0  0  0  0  0  0  0  0  0  0  0  0  0  0; 0  0  0  0  0  0  0  0  0  0  0  0  0  0  0  0  0  0  0  0  0; 0  0  0  0  0  0  0  0  0  0  0  0  0  0  0  0  0  0  0  0  0; 0  0  0  0  0  0  0  0  0  0  0  0  0  0  0  0  0  0  0  0  0; 0  0  0  0  0  0  0  0  0  0  0  0  0  0  0  0  0  0  0  0  0; 0  0  0  0  0  0  0  0  0  0  0  0  0  0  0  0  0  0  0  0  0; 0  0  0  0  0  0  0  0  0  0  0  0  0  0  0  0  0  0  0  0  0; 0  0  0  0  0  0  0  0  0  0  0  0  0  0  0  0  0  0  0  0  0; 0  0  0  0  0  0  0  0  0  0  0  0  0  0  0  0  0  0  0  0  0; 0  0  0  0  0  0  0  0  0  0  0  0  0  0  0  0  0  0  0  0  0; 0  0  0  0  0  0  0  0  0  0  0  0  0  0  0  0  0  0  0  0  0; 0  0  0  0  0  0  0  0  0  0  0  0  0  0  0  0  0  0  0  0  0; 0  0  0  0  0  0  0  0  0  0  0  0  0  0  0  0  0  0  0  0  0; 0  0  0  0  0  0  0  0  0  0  0  0  0  0  0  0  0  0  0  0  0; 0  0  0  0  0  0  0  0  0  0  0  0  0  0  0  0  0  0  0  0  0; 0  0  0  0  0  0  0  0  0  0  0  0  0  0  0  0  0  0  0  0  0]
  f_sa = [9.05 9.05 16.4373253582 15.3405265461 13.6074880273 9.83352189562 3.89388784387 0 0 0 0 0 ... (240 elements, 16x15)]
  f_sa_ld_bpt = [0 0.2 0.275 0.35 0.425 0.5 0.575 0.65 0.725 0.8 0.875 0.95 1.025 1.1 1.175 1.25]
  f_sa_n_bpt = [750 1053.57142857 1357.14285714 1660.71428571 1964.28571429 2267.85714286 2571.42857143 2875 3178.57142857 3482.14285714 3785.71428571 4089.28571429 4392.85714286 4696.42857143 5000]
  f_sa_opt = [35.3085 21.0105 10.3714 8.5076 7.1426 7.5656 -5.7766 -16.7061 -16.8345 -19.3546 -20.6085 -22.0872 ... (225 elements, 15x15)]
  f_startup_ect_bpt = [-40 0 20 50]
  f_startup_lambda_delta = [0.5 0.3 0.2 0]
  f_startup_lambda_delta_timecnst = [90 40 12 0]
  f_susp_axl_bp = [1 2]
  f_susp_dz_bp = [-0.325022776267 -0.315022776267 -0.305022776267 -0.205022776267 -0.105022776267 -0.00502277626717 0.0949772237328 0.194977223733 0.204977223733 0.214977223733]
  f_susp_dzdot_bp = [-3 -0.3 -0.2 -0.1 0 0.1 0.2 0.3 3]
  f_susp_fmz = [-144070.391448 -93629.24037 -75929.1118915 -20630.5828179 -15385.48216 -10140.3815021 -4895.28084414 349.819813785 -31916.3973792 18437.6709544 -83996.1993354 -33555.0482577 ... (43920 elements, 10x9x61x2x4)]
  f_susp_geom = [0 0 0 0 0 0 0 0 0 0 0 0 ... (3660 elements, 10x61x2x3)]
  f_susp_strgdelta_bp = [-0.523598775598 -0.506145483078 -0.488692190558 -0.471238898038 -0.453785605519 -0.436332312999 -0.418879020479 -0.401425727959 -0.383972435439 -0.366519142919 -0.349065850399 -0.331612557879 -0.314159265359 -0.296705972839 -0.279252680319 -0.261799387799 -0.244346095279 -0.226892802759 -0.209439510239 -0.191986217719 -0.174532925199 -0.157079632679 -0.13962634016 -0.12217304764 -0.10471975512 -0.0872664625997 -0.0698131700798 -0.0523598775598 -0.0349065850399 -0.0174532925199 0 0.0174532925199 0.0349065850399 0.0523598775598 0.0698131700798 0.0872664625997 0.10471975512 0.12217304764 0.13962634016 0.157079632679 0.174532925199 0.191986217719 0.209439510239 0.226892802759 0.244346095279 0.261799387799 0.279252680319 0.296705972839 0.314159265359 0.331612557879 0.349065850399 0.366519142919 0.383972435439 0.401425727959 0.418879020479 0.436332312999 0.453785605519 0.471238898038 0.488692190558 0.506145483078 0.523598775598]
  f_t_exh = [739.936218766 750.584766028 772.770773797 791.235245621 803.106549716 885.862998064 920.498479307 920.498479307 920.498479307 920.498479307 920.498479307 920.498479307 ... (225 elements, 15x15)]
  f_t_exh_l_bpt = [0.2 0.275 0.35 0.425 0.5 0.575 0.65 0.725 0.8 0.875 0.95 1.025 1.1 1.175 1.25]
  f_t_exh_n_bpt = [750 1053.57142857 1357.14285714 1660.71428571 1964.28571429 2267.85714286 2571.42857143 2875 3178.57142857 3482.14285714 3785.71428571 4089.28571429 4392.85714286 4696.42857143 5000]
  f_tap = [0 0.9375 0.9375 0.982121188204 1.22093639741 1.5421156717 1.98870690459 2.59666257968 2.6875 2.6875 2.6875 2.6875 ... (315 elements, 21x15)]
  f_tap_ld_bpt = [0 0.2 0.268421052632 0.336842105263 0.405263157895 0.473684210526 0.542105263158 0.610526315789 0.678947368421 0.747368421053 0.815789473684 0.884210526316 0.952631578947 1.02105263158 1.08947368421 1.15789473684 1.22631578947 1.29473684211 1.36315789474 1.43157894737 1.5]
  f_tap_n_bpt = [750 1053.57142857 1357.14285714 1660.71428571 1964.28571429 2267.85714286 2571.42857143 2875 3178.57142857 3482.14285714 3785.71428571 4089.28571429 4392.85714286 4696.42857143 5000]
  f_tbrake = [0 10.8721902117 10.8721902117 10.8721902117 10.8721902117 10.8721902117 10.8721902117 10.8721902117 10.8721902117 10.8721902117 10.8721902117 10.8721902117 ... (441 elements, 21x21)]
  f_tbrake_n_bpt = [0 750 973.684210526 1197.36842105 1421.05263158 1644.73684211 1868.42105263 2092.10526316 2315.78947368 2539.47368421 2763.15789474 2986.84210526 3210.52631579 3434.21052632 3657.89473684 3881.57894737 4105.26315789 4328.94736842 4552.63157895 4776.31578947 5000]
  f_tbrake_t_bpt = [0; 16.186104388; 24.9146526824; 33.6432009767; 42.3717492711; 51.1002975655; 59.8288458599; 68.5573941543; 77.2859424487; 86.0144907431; 94.7430390375; 103.471587332; 112.200135626; 120.928683921; 129.657232215; 138.385780509; 147.114328804; 155.842877098; 164.571425393; 173.299973687; 182.028521981]
  f_texh = [630.359790352 638.212816583 644.85156876 656.410931683 676.180276582 706.880985433 749.880156186 804.757804763 869.00210738 938.264388175 1007.38061415 1071.70023123 ... (441 elements, 21x21)]
  f_tm_corr = [0.839360054391 0.833393271885 0.82629554201 0.818442814437 0.811524387436 0.809164184856 0.814606352881 0.826887956871 0.842304598924 0.856886829014 0.869487025783 0.880530414174 ... (400 elements, 20x20)]
  f_tm_corr_n_bpt = [750 973.6842 1197.3684 1421.0526 1644.7368 1868.4211 2092.1053 2315.7895 2539.4737 2763.1579 2986.8421 3210.5263 3434.2105 3657.8947 3881.5789 4105.2632 4328.9474 4552.6316 4776.3158 5000]
  f_tm_corr_nd_bpt = [0.3 0.38947 0.47895 0.56842 0.65789 0.74737 0.83684 0.92632 1.0158 1.1053 1.1947 1.2842 1.3737 1.4632 1.5526 1.6421 1.7316 1.8211 1.9105 2]
  f_tpp = [0 100]
  f_tpp_tap_bpt = [0 100]
  f_tq_fric = [4.16  4.8  5.44  6.05  6.64  7.23  7.81  8.39  8.97  9.54  10.1  10.7  11.3  11.9  12.5; 4.42  5.07  5.69  6.29  6.89  7.49  8.09  8.69  9.28  9.86  10.4  11  11.6  12.2  12.8; 4.69  5.36  5.98  6.58  7.18  7.79  8.41  9.02  9.62  10.2  10.8  11.4  11.9  12.5  13.1; 4.88  5.59  6.25  6.87  7.48  8.09  8.71  9.32  9.92  10.5  11.1  11.7  12.3  12.9  13.4; 4.94  5.74  6.45  7.12  7.75  8.37  8.99  9.59  10.2  10.8  11.4  11.9  12.6  13.2  13.8; 4.93  5.76  6.56  7.29  7.97  8.62  9.23  9.83  10.4  11  11.6  12.2  12.8  13.4  14.1; 4.85  5.67  6.57  7.37  8.11  8.8  9.43  10  10.6  11.2  11.8  12.4  13  13.7  14.3; 4.74  5.57  6.46  7.34  8.14  8.88  9.55  10.2  10.8  11.4  12  12.6  13.2  13.8  14.4; 4.63  5.42  6.27  7.19  8.05  8.83  9.55  10.2  10.9  11.5  12.1  12.7  13.3  14  14.6; 4.52  5.29  6.11  6.98  7.84  8.65  9.4  10.1  10.8  11.5  12.1  12.8  13.4  14.1  14.6; 4.42  5.18  5.97  6.79  7.6  8.39  9.15  9.88  10.6  11.3  12.1  12.8  13.5  14.1  14.7; 4.34  5.09  5.86  6.64  7.42  8.17  8.88  9.6  10.3  11.1  11.9  12.7  13.4  14.1  14.7; 4.27  5.01  5.76  6.52  7.28  8.03  8.74  9.39  10.1  10.8  11.6  12.4  13.2  14  14.7; 4.21  4.94  5.67  6.42  7.16  7.89  8.59  9.25  9.93  10.7  11.5  12.3  13.1  13.8  14.6; 4.15  4.87  5.6  6.33  7.06  7.77  8.47  9.14  9.84  10.6  11.3  12.1  12.9  13.7  14.4]
  f_tq_inr = [25.8508 37.8267 50.6081 62.6825 74.6026 88.9064 81.9508 76.6399 82.9886 85.0042 88.9209 92.7645 ... (225 elements, 15x15)]
  f_tq_inr_l_bpt = [0.2 0.28571 0.37143 0.45714 0.54286 0.62857 0.71429 0.8 0.88571 0.97143 1.0571 1.1429 1.2286 1.3143 1.4]
  f_tq_inr_n_bpt = [750 1053.5714 1357.1429 1660.7143 1964.2857 2267.8571 2571.4286 2875 3178.5714 3482.1429 3785.7143 4089.2857 4392.8571 4696.4286 5000]
  f_tq_nl = [0 15.0012133443 26.4298333923 37.8556656512 49.2846782956 60.7113978793 72.3451969202 77.459652163 78.5324534074 78.5324534074 78.5324534074 78.5324534074 ... (256 elements, 16x16)]
  f_tq_nl_l_bpt = [0 0.2 0.275 0.35 0.425 0.5 0.575 0.65 0.725 0.8 0.875 0.95 1.025 1.1 1.175 1.25]
  f_tq_nl_n_bpt = [0 750 1053.57142857 1357.14285714 1660.71428571 1964.28571429 2267.85714286 2571.42857143 2875 3178.57142857 3482.14285714 3785.71428571 4089.28571429 4392.85714286 4696.42857143 5000]
  f_tq_pump = [7.24  7.7  7.82  7.95  8.1  8.27  8.45  8.64  8.78  8.88  8.96  9.03  9.12  9.25  9.45; 5.67  6.03  6.37  6.67  6.92  7.14  7.33  7.5  7.67  7.84  8.01  8.19  8.38  8.58  8.8; 3.94  4.52  5  5.36  5.6  5.77  5.92  6.1  6.35  6.67  7.02  7.4  7.75  8.06  8.34; 2.59  3.14  3.57  3.86  4.05  4.21  4.43  4.76  5.21  5.75  6.32  6.85  7.3  7.65  7.92; 1.8  2.25  2.61  2.88  3.11  3.37  3.71  4.17  4.74  5.36  5.96  6.49  6.91  7.23  7.46; 1  1.36  1.77  2.15  2.51  2.88  3.31  3.8  4.37  4.98  5.57  6.11  6.57  6.94  7.25; 1  1  1  1.09  1.59  2.08  2.6  3.17  3.81  4.49  5.19  5.85  6.44  6.92  7.29; 1  1  1  1  1  1.62  2.32  3.05  3.83  4.64  5.44  6.19  6.82  7.31  7.65; 1  1  1  1  1  1.35  2.21  3.08  3.97  4.88  5.78  6.64  7.41  8.06  8.58; 1  1  1  1  1  1  1.77  2.67  3.58  4.55  5.6  6.73  7.91  9.07  10.1; 1  1  1  1  1  1  1.72  2.67  3.61  4.62  5.79  7.15  8.69  10.3  11.9; 1  1  1  1  1  1  1.74  2.88  3.96  5.08  6.36  7.86  9.57  11.4  13.2; 1  1  1  1  1  1  1.37  2.7  4.01  5.39  6.92  8.65  10.5  12.4  14.2; 1  1  1  1  1  1  1.28  2.66  4.14  5.72  7.43  9.28  11.2  13.1  14.8; 1  1  1  1  1  1  1.39  2.82  4.39  6.06  7.85  9.73  11.6  13.5  15.1]
  f_twc_eff_co = [0.17 0.25 0.45 0.99 0.99 0.99 0.99]
  f_twc_eff_hc = [0.21 0.375 0.75 0.98 0.98 0.98 0.98]
  f_twc_eff_lam = [0.909090909 0.944055944 0.979020979 1 1.013986014 1.048951049 1.083916084]
  f_twc_eff_nox = [0.98 0.98 0.98 0.97 0.05 0.02 0]
  f_vivc = [0.37716 0.38164 0.38611 0.39033 0.39428 0.39795 0.40132 0.40441 0.40719 0.40967 0.41184 0.41372 0.41529 0.41656 0.41755 0.41825 0.41867 0.41884 0.41874 0.41865]
  f_vivc_icp_bpt = [0 2.6316 5.2632 7.8947 10.5263 13.1579 15.7895 18.4211 21.0526 23.6842 26.3158 28.9474 31.5789 34.2105 36.8421 39.4737 42.1053 44.7368 47.3684 50]
  f_wap = [100 100 100 100 100 100 100 99.9999999843 99.9999999843 99.9999999843 99.9999999843 99.9999999843 ... (315 elements, 21x15)]
  f_wap_ld_bpt = [0 0.2 0.268421052632 0.336842105263 0.405263157895 0.473684210526 0.542105263158 0.610526315789 0.678947368421 0.747368421053 0.815789473684 0.884210526316 0.952631578947 1.02105263158 1.08947368421 1.15789473684 1.22631578947 1.29473684211 1.36315789474 1.43157894737 1.5]
  f_wap_n_bpt = [750 1053.57142857 1357.14285714 1660.71428571 1964.28571429 2267.85714286 2571.42857143 2875 3178.57142857 3482.14285714 3785.71428571 4089.28571429 4392.85714286 4696.42857143 5000]
  g = 9.81
  h = 0.134
  k = Simulink.Parameter
  k.Value = 10000
  k.DataType = 'auto'
  k.Dimensions = [1 1]
  k1 = 50000
  k2 = 50000
  kappamax = 1.5
  lam_x = 1
  maxAccel = 3
  maxVel = 20
  minAccel = -3
  mu_kinetic = 0.35
  mu_static = 0.45
  muc = [0.16 0.13 0.115 0.11 0.105 0.1025 0.10125]
  muk = 0.4
  mus = 0.45
  numWheel = 4
  num_pads = 2
  omega1_c = 3000
  omega2_c = 3000
  omega_bpts = [52.4 78.5 105 131 157 183 209 262 314 419 524]
  omega_c = Simulink.Parameter
  omega_c.Value = 500
  omega_c.DataType = 'auto'
  omega_c.Dimensions = [1 1]
  omega_o = 0
  omega_o_J = 0
  omegai_o = 0
  omegain_o = 0
  omegal = 94.2477796077
  omegao = 0
  omegaout_o = 0
  omegat_o = 0
  omegau = 83.7758040957
  omegaw1o = 0
  omegaw2o = 0
  phi = [0 0.5 0.6 0.7 0.8 0.87 0.92 0.94 0.96 0.97]
  philu = 0.85
  power_max = 30000
  predHorizon = 300
  press = 234400
  psi = [12.2938 12.8588 13.1452 13.6285 14.6163 16.2675 19.3503 22.1046 29.9986 50]
  q_o = 0
  sampleTime = 0.01
  stopTime = 1000000
  switchDist = 200
  switchVel = 0
  tauC = 0.6
  tauC_1 = 0.1
  tauC_LSD = 0.01
  tauTC = 0.1
  tau_egr = 0.2
  tau_s = 0.08
  tc = 0.01
  theta_o = 0
  theta_o_Veh = 0
  time_gap = 1
  torque_max = 200
  ts = 0.01
  v_0 = 0
  v_set = 10
  w1_o = 0
  w_eff_bp = [0 500 1000 1432.391138 1500 2000 2500 3000 3500 4000 4500 5000 5500 6000]
  w_eff_bp_EV_front = [0 1666.66666667 3333.33333333 4774.63712667 5000 6666.66666667 8333.33333333 10000 11666.6666667 13333.3333333 15000 16666.6666667 18333.3333333 20000]
  w_eff_bp_EV_rear = [0 1666.66666667 3333.33333333 4774.63712667 5000 6666.66666667 8333.33333333 10000 11666.6666667 13333.3333333 15000 16666.6666667 18333.3333333 20000]
  w_eff_bp_P0 = [0 500 1000 1432.39448783 4500 6000 7500 9000 10500 12000 13500 15000 16500 18000]
  wc = 10
  win_o = 0
  wout_o = 0
  x_o = 0
  xdot_o = 0
  z_o = -0.35
  zdot_o = 0
  zeta = [2.232 1.5462 1.4058 1.2746 1.1528 1.0732 1.0192 0.9983 0.9983 0.9983]
undefined symbols (not defined in the file or in its folder): Disabled, DLCXref, DLCYref, Right, sigbuilder_block, SRE
libraries: simulink x11, vehdynlibscenariocommon x5, simulink_extras x5, vrlib x2, sim3dlib x2, vehdynlibviscommon x2, autolibshared x1, vehdynlibdriver x1, sim3dautolib x1
(part 1 of 6)
settings Model: DataDictionary=System_Data_Dictionary.sldd  ModifiedByFormat=The MathWorks, Inc.  PauseTimes=23.46  OrderedModelArguments=off  Creator=The MathWorks, Inc.  LastModifiedBy=The MathWorks, Inc.
settings ConfigSetRef: SourceName=Config_VarStep_Lat

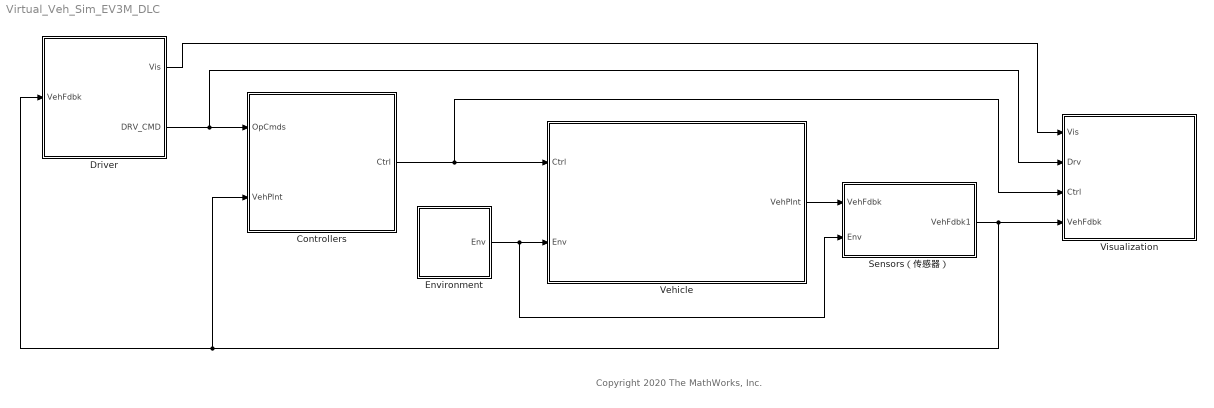
== system Virtual_Veh_Sim_EV3M_DLC ==
  note: Copyright 2020 The MathWorks, Inc.
  Controllers : Subsystem
      mask Display: image('SystemControllers.png', 'center')
  Driver : Subsystem  Variant=on  VariantControlMode=Label  LabelModeActiveChoice=2
  Environment : Subsystem  VariantControl=2
      mask Display: disp('Environment')
  Sensors（传感器） : Subsystem  Variant=on  VariantControlMode=Label  VariantControl=Variant1  LabelModeActiveChoice=0
  Vehicle : Subsystem
      mask Display: image('PassengerVehicle.png', 'center')
  Visualization : Subsystem  Variant=on  VariantControlMode=Label  LabelModeActiveChoice=2
  wires:
  Environment/1(Env) -> Vehicle/2(Env), Sensors（传感器）/2(Env)
  Controllers/1(Ctrl) -> Visualization/3(Ctrl), Vehicle/1(Ctrl)
  Driver/2(DRV_CMD) -> Visualization/2(Drv), Controllers/1(OpCmds)
  Vehicle/1(VehPlnt) -> Sensors（传感器）/1(VehFdbk)
  Driver/1(Vis) -> Visualization/1(Vis)
  Sensors（传感器）/1(VehFdbk1) -> Visualization/4(VehFdbk), Driver/1(VehFdbk), Controllers/2(VehPlnt)
